simulink model "arx_oe_ex1"  (Simulink 5.0)
settings: Solver=ode45  StartTime=0.0  StopTime=3999  RelTol=1e-3
settings Model: Creator=akt1  LastModifiedBy=aruntangirala  ExtModeAutoUpdateStatusClock=off  BlockReductionOpt=off  BooleanDataType=off

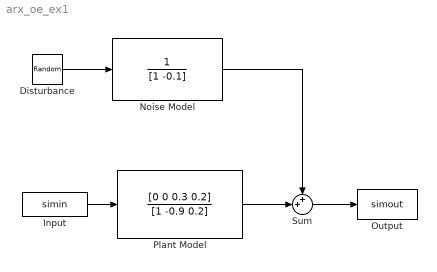
== system arx_oe_ex1 ==
  Disturbance : RandomNumber  Variance=0.2  SampleTime=0
  Input : FromWorkspace  VariableName=simin  SampleTime=0
  Noise Model : DiscreteFilter  Numerator=1  Denominator=[1 -0.1]
  Output : ToWorkspace  VariableName=simout  SampleTime=-1  SaveFormat=Array
  Plant Model : DiscreteFilter  Numerator=[0 0 0.3 0.2]  Denominator=[1 -0.9 0.2]
  Sum : Sum  Inputs=++|  SaturateOnIntegerOverflow=on  InputSameDT=on
  wires:
  Input/1 -> Plant Model/1
  Disturbance/1 -> Noise Model/1
  Plant Model/1 -> Sum/2
  Noise Model/1 -> Sum/1
  Sum/1 -> Output/1
